simulink model "shuangxiangkaiguan"  (R2016b)
settings: Solver=ode23t  StartTime=0.0  StopTime=0.5  RelTol=1e-3
libraries: powerlib x31
settings Model: Creator=ChenNingke  LastModifiedBy=CNK

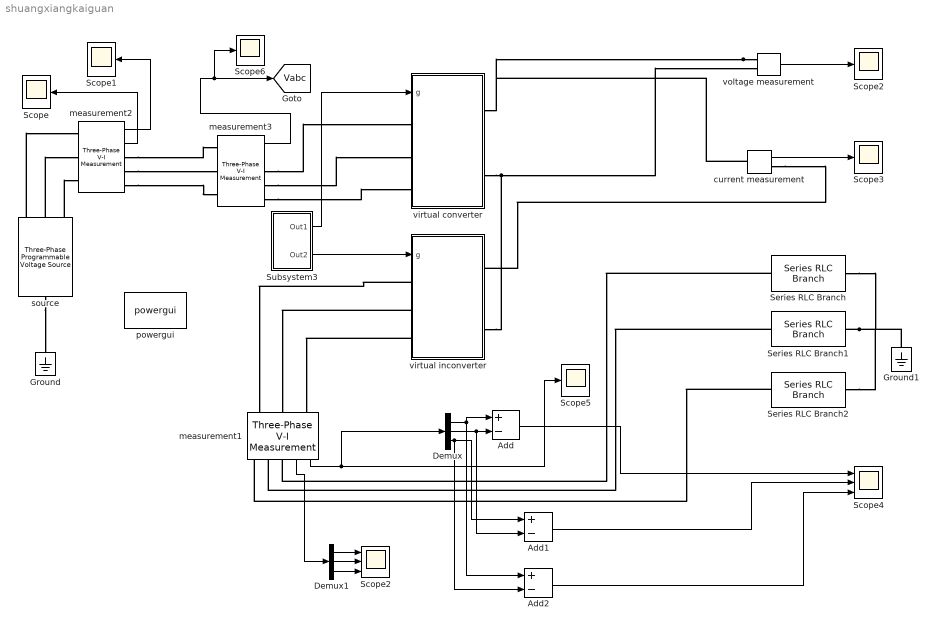
== system shuangxiangkaiguan ==
  Add : Sum  Inputs=+-
  Add1 : Sum  Inputs=+-
  Add2 : Sum  Inputs=+-
  Demux : Demux  Outputs=3
  Demux1 : Demux  Outputs=3
  Ground : powerlib/Elements/Ground  LConnTagsString=a
  Ground1 : powerlib/Elements/Ground  LConnTagsString=a
  Scope{,1,3,5..6} (5 alike) : Scope
  Scope2 : Scope  NumInputPorts=3
  "Scope2 " : Scope
  Scope4 : Scope  NumInputPorts=3
  Series RLC Branch : powerlib/Elements/Series RLC Branch  LConnTagsString=__new0  RConnTagsString=__new0  BranchType=RL  Resistance=5  Inductance=5e-3  SetiL0=off  InitialCurrent=0  Capacitance=1e-6  Setx0=off  InitialVoltage=0  Measurements=None
  Series RLC Branch1 : powerlib/Elements/Series RLC Branch  LConnTagsString=__new0  RConnTagsString=__new0  BranchType=RL  Resistance=5  Inductance=5e-3  SetiL0=off  InitialCurrent=0  Capacitance=1e-6  Setx0=off  InitialVoltage=0  Measurements=None
  Series RLC Branch2 : powerlib/Elements/Series RLC Branch  LConnTagsString=__new0  RConnTagsString=__new0  BranchType=RL  Resistance=5  Inductance=5e-3  SetiL0=off  InitialCurrent=0  Capacitance=1e-6  Setx0=off  InitialVoltage=0  Measurements=None
  Subsystem3 : Subsystem
  current measurement : powerlib/Measurements/Current Measurement  PhasorSimulation=off  OutputType=Complex  PSBequivalent=0
  measurement1 : powerlib/Measurements/Three-Phase V-I Measurement  VoltageMeasurement=phase-to-phase  SetLabelV=off  LabelV=Vabc  Vpu=off  VpuLL=off  CurrentMeasurement=yes  SetLabelI=off  LabelI=Iabc  Ipu=off  Pbase=100e6  Vbase=500e3  OutputType=Complex  PhasorSimulation=off  PSBequivalent=0
  measurement2 : powerlib/Measurements/Three-Phase V-I Measurement  VoltageMeasurement=phase-to-phase  SetLabelV=off  LabelV=Vabc  Vpu=off  VpuLL=off  CurrentMeasurement=yes  SetLabelI=off  LabelI=Iabc  Ipu=off  Pbase=100e6  Vbase=500e3  OutputType=Complex  PhasorSimulation=off  PSBequivalent=0
  measurement3 : powerlib/Measurements/Three-Phase V-I Measurement  VoltageMeasurement=phase-to-phase  SetLabelV=off  LabelV=Vabc  Vpu=off  VpuLL=off  CurrentMeasurement=yes  SetLabelI=off  LabelI=Iabc  Ipu=off  Pbase=100e6  Vbase=500e3  OutputType=Complex  PhasorSimulation=off  PSBequivalent=0
  powergui : powerlib/powergui  Priority=1  SimulationMode=Continuous  SolverType=Tustin  SampleTime=50e-6  frequency=60  SPID=off  DisableSnubberDevices=off  DisableRonSwitches=off  DisableVfSwitches=off  SwTol=0  DisplayEquations=off  Interpol=off  ExternalGateDelay=off  methode=off  Ts=10  FunctionMessages=off  echomessages=off  HookPort=off  EnableUseOfTLC=off  x0status=blocks  frequencyindice=0  Pbase=100e6  ErrMax=1e-4  Iterations=50  UnitsV=kV  UnitsW=MW  buscounter=0  RestoreLinks=warning  ResistiveCurrentMeasurement=off  Frange=[0:2:500]  Ylog=off  Xlog=on  ShowGrid=off  save=off  variable=ZData  structure=ScopeData6  ZoomFFT=off  StartTime=0.0  cycles=1  DisplayStyle=1  fundamental=600  FreqAxis=off  MaxFrequency=2000  frequencyindicesteady=1  RmsSteady=1  display=off
  source : powerlib/Electrical Sources/Three-Phase Programmable Voltage Source  PositiveSequence="[220  0 50]"  VariationEntity=None  VariationType=Table of time-amplitude pairs  VariationTypeAlt=Step  VariationStep=0.5  VariationRate=10  VariationMagnitude=0.3  VariationFrequency=2  VariationTiming=[1 2]  VariationPhaseA=off  Amplitudes=[1 0.8 1.2 1.0]  TimeValues=[0 0.1 0.15 0.2]  HarmonicGeneration=off  HarmonicA=[3 0.2 -25 0]  HarmonicB=[2 0.15 35 2]  Timing="[0.05  3]"  BusType=swing  Pref=0  Qref=0  Qmin=-inf  Qmax=inf
  virtual converter : Subsystem
  virtual inconverter : Subsystem
  voltage measurement : powerlib/Measurements/Voltage Measurement  PhasorSimulation=off  OutputType=Complex  PSBequivalent=0
  tag scope: Vabc=global
  wires:
  voltage measurement/1 -> "Scope2 "/1
  current measurement/1 -> Scope3/1
  measurement2/2 -> Scope/1
  measurement1/1 -> Demux/1, Scope5/1
  Subsystem3/2(Out2) -> virtual inconverter/1(g)
  Subsystem3/1(Out1) -> virtual converter/1(g)
  measurement2/1 -> Scope1/1
  Demux/1 -> Add2/1, Add/1
  Demux/2 -> Add1/2, Add/2
  Add/1 -> Scope4/1
  Demux/3 -> Add2/2, Add1/1
  Add1/1 -> Scope4/2
  Add2/1 -> Scope4/3
  measurement1/2 -> Demux1/1
  Demux1/1 -> Scope2/1
  Demux1/2 -> Scope2/2
  Demux1/3 -> Scope2/3
  measurement3/1 -> [Vabc], Scope6/1
  connections:
  voltage measurement/LConn1 -- current measurement/LConn1 -- virtual converter/RConn1
  virtual converter/RConn2 -- virtual inconverter/RConn2 -- voltage measurement/LConn2
  Series RLC Branch1/RConn1 -- Ground1/LConn1 -- Series RLC Branch/RConn1 -- Series RLC Branch2/RConn1
  Series RLC Branch1/LConn1 -- measurement1/RConn2
  current measurement/RConn1 -- virtual inconverter/RConn1
  Series RLC Branch/LConn1 -- measurement1/RConn1
  Series RLC Branch2/LConn1 -- measurement1/RConn3
  source/LConn1 -- Ground/LConn1
  virtual inconverter/LConn1 -- measurement1/LConn3
  virtual inconverter/LConn2 -- measurement1/LConn2
  virtual inconverter/LConn3 -- measurement1/LConn1
  source/RConn1 -- measurement2/LConn1
  source/RConn2 -- measurement2/LConn2
  source/RConn3 -- measurement2/LConn3
  measurement2/RConn1 -- measurement3/LConn1
  measurement2/RConn2 -- measurement3/LConn2
  measurement2/RConn3 -- measurement3/LConn3
  measurement3/RConn3 -- virtual converter/LConn3
  measurement3/RConn2 -- virtual converter/LConn2
  measurement3/RConn1 -- virtual converter/LConn1

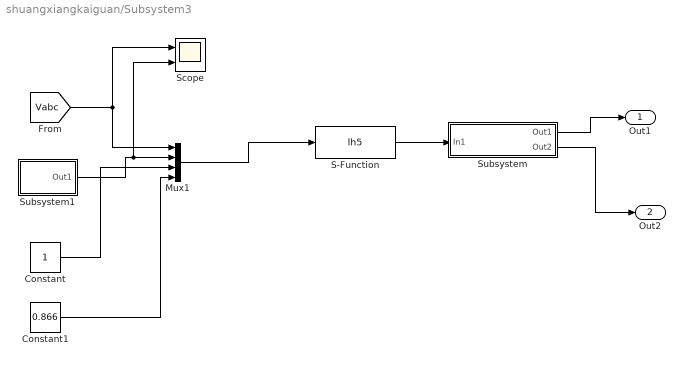
== system shuangxiangkaiguan/Subsystem3 ==
  Constant : Constant
  Constant1 : Constant  Value=0.866
  Mux1 : Mux
  S-Function : S-Function  FunctionName=lh5  SFunctionDeploymentMode=off  EnableBusSupport=off
  Scope : Scope  NumInputPorts=2
  Subsystem : Subsystem
  Subsystem1 : Subsystem
  Out1 : Outport
  Out2 : Outport  Port=2
  wires:
  [Vabc] -> Scope/1, Mux1/1
  Subsystem/1(Out1) -> Out1/1
  S-Function/1 -> Subsystem/1(In1)
  Subsystem1/1(Out1) -> Scope/2, Mux1/2
  Constant1/1 -> Mux1/4
  Constant/1 -> Mux1/3
  Subsystem/2(Out2) -> Out2/1
  Mux1/1 -> S-Function/1

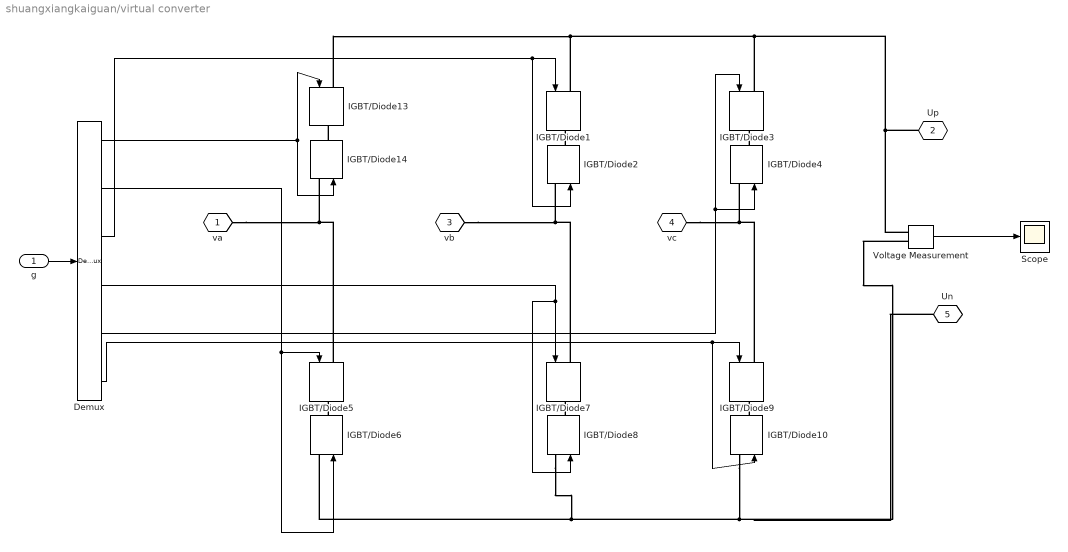
== system shuangxiangkaiguan/virtual converter ==
  g : Inport
  Demux : Demux  Outputs=6
  IGBT/Diode{1..10,13..14} (12 alike) : powerlib/Power Electronics/IGBT//Diode  Ron=1e-3  Rs=1e5  Cs=inf  Measurements=off
  Scope : Scope
  Voltage Measurement : powerlib/Measurements/Voltage Measurement  PhasorSimulation=off  OutputType=Complex  PSBequivalent=0
  va : PMIOPort  Tag=PMCPort  Port=1  Side=Left
  Up : PMIOPort  Tag=PMCPort  Port=2  Side=Right
  vb : PMIOPort  Tag=PMCPort  Port=3  Side=Left
  vc : PMIOPort  Tag=PMCPort  Port=4  Side=Left
  Un : PMIOPort  Tag=PMCPort  Port=5  Side=Right
  wires:
  g/1 -> Demux/1
  Demux/1 -> IGBT/Diode13/1, IGBT/Diode14/1
  Demux/3 -> IGBT/Diode1/1, IGBT/Diode2/1
  Demux/5 -> IGBT/Diode4/1, IGBT/Diode3/1
  Voltage Measurement/1 -> Scope/1
  Demux/2 -> IGBT/Diode5/1, IGBT/Diode6/1
  Demux/4 -> IGBT/Diode8/1, IGBT/Diode7/1
  Demux/6 -> IGBT/Diode10/1, IGBT/Diode9/1
  connections:
  va/RConn1 -- IGBT/Diode5/LConn1 -- IGBT/Diode14/LConn1
  vb/RConn1 -- IGBT/Diode7/LConn1 -- IGBT/Diode2/LConn1
  vc/RConn1 -- IGBT/Diode9/LConn1 -- IGBT/Diode4/LConn1
  Up/RConn1 -- Voltage Measurement/LConn1 -- IGBT/Diode1/LConn1 -- IGBT/Diode13/LConn1 -- IGBT/Diode3/LConn1
  Voltage Measurement/LConn2 -- Un/RConn1 -- IGBT/Diode10/LConn1 -- IGBT/Diode6/LConn1 -- IGBT/Diode8/LConn1
  IGBT/Diode14/RConn1 -- IGBT/Diode13/RConn1
  IGBT/Diode2/RConn1 -- IGBT/Diode1/RConn1
  IGBT/Diode4/RConn1 -- IGBT/Diode3/RConn1
  IGBT/Diode6/RConn1 -- IGBT/Diode5/RConn1
  IGBT/Diode8/RConn1 -- IGBT/Diode7/RConn1
  IGBT/Diode10/RConn1 -- IGBT/Diode9/RConn1

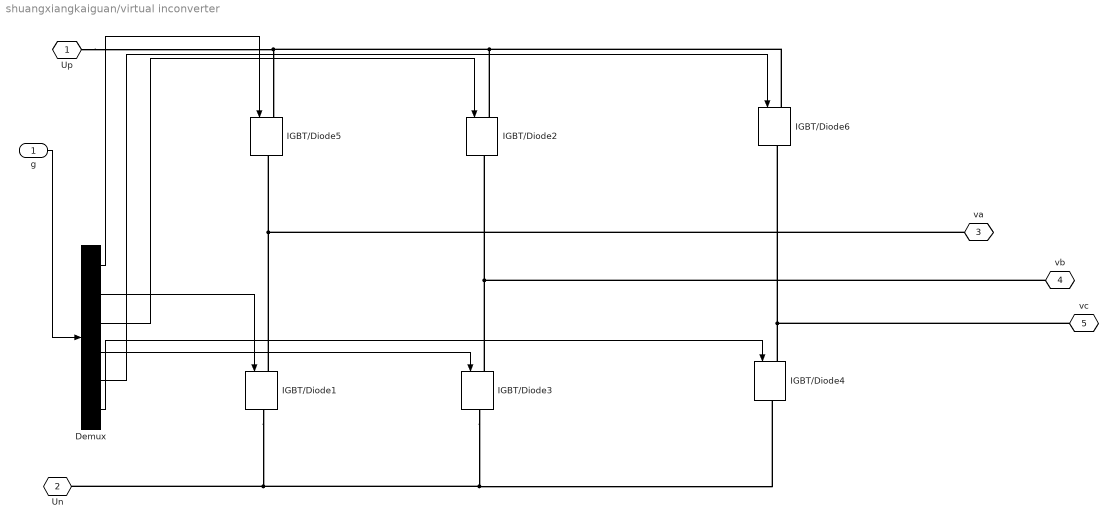
== system shuangxiangkaiguan/virtual inconverter ==
  g : Inport
  Demux : Demux  Outputs=6
  IGBT/Diode{1..6} (6 alike) : powerlib/Power Electronics/IGBT//Diode  Ron=1e-3  Rs=1e5  Cs=inf  Measurements=off
  Up : PMIOPort  Tag=PMCPort  Port=1  Side=Right
  Un : PMIOPort  Tag=PMCPort  Port=2  Side=Right
  va : PMIOPort  Tag=PMCPort  Port=3  Side=Left
  vb : PMIOPort  Tag=PMCPort  Port=4  Side=Left
  vc : PMIOPort  Tag=PMCPort  Port=5  Side=Left
  wires:
  g/1 -> Demux/1
  Demux/1 -> IGBT/Diode5/1
  Demux/3 -> IGBT/Diode2/1
  Demux/5 -> IGBT/Diode6/1
  Demux/6 -> IGBT/Diode4/1
  Demux/2 -> IGBT/Diode1/1
  Demux/4 -> IGBT/Diode3/1
  connections:
  vc/RConn1 -- IGBT/Diode6/RConn1 -- IGBT/Diode4/LConn1
  vb/RConn1 -- IGBT/Diode2/RConn1 -- IGBT/Diode3/LConn1
  va/RConn1 -- IGBT/Diode1/LConn1 -- IGBT/Diode5/RConn1
  Up/RConn1 -- IGBT/Diode2/LConn1 -- IGBT/Diode6/LConn1 -- IGBT/Diode5/LConn1
  Un/RConn1 -- IGBT/Diode4/RConn1 -- IGBT/Diode3/RConn1 -- IGBT/Diode1/RConn1

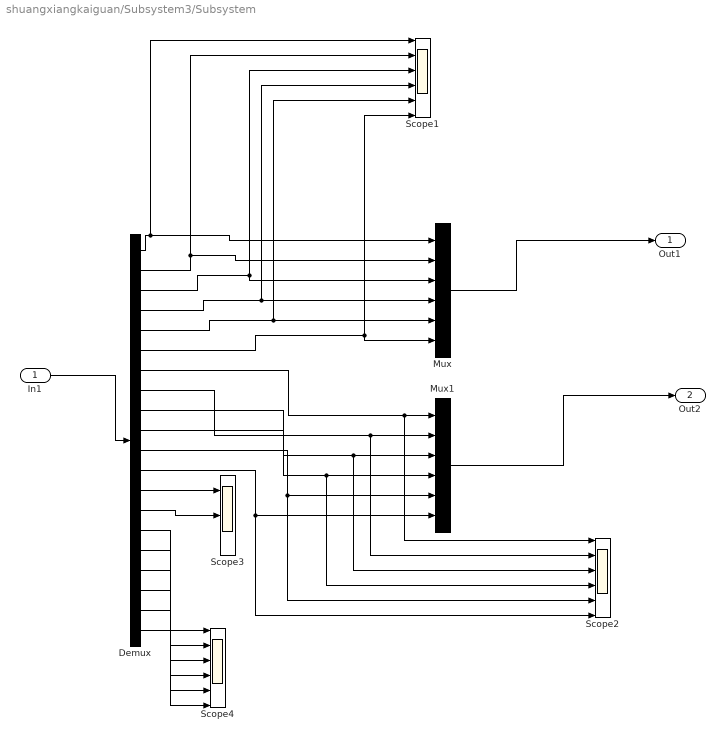
== system shuangxiangkaiguan/Subsystem3/Subsystem ==
  In1 : Inport
  Demux : Demux  Outputs=20
  Mux : Mux  Inputs=6
  Mux1 : Mux  Inputs=6
  Scope1 : Scope  NumInputPorts=6
  Scope2 : Scope  NumInputPorts=6
  Scope3 : Scope  NumInputPorts=3
  Scope4 : Scope  NumInputPorts=6
  Out1 : Outport
  Out2 : Outport  Port=2
  wires:
  In1/1 -> Demux/1
  Demux/1 -> Mux/1, Scope1/1
  Demux/2 -> Mux/2, Scope1/2
  Demux/3 -> Mux/3, Scope1/3
  Demux/4 -> Scope1/4, Mux/4
  Demux/5 -> Scope1/5, Mux/5
  Mux/1 -> Out1/1
  Demux/6 -> Mux/6, Scope1/6
  Demux/7 -> Scope2/1, Mux1/1
  Demux/8 -> Scope2/2, Mux1/2
  Demux/9 -> Scope2/3, Mux1/3
  Demux/10 -> Scope2/4, Mux1/4
  Demux/11 -> Scope2/5, Mux1/5
  Demux/12 -> Scope2/6, Mux1/6
  Mux1/1 -> Out2/1
  Demux/13 -> Scope3/1
  Demux/14 -> Scope3/2
  Demux/15 -> Scope4/1
  Demux/16 -> Scope4/2
  Demux/17 -> Scope4/3
  Demux/18 -> Scope4/4
  Demux/19 -> Scope4/5
  Demux/20 -> Scope4/6

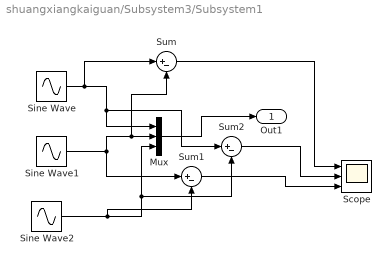
== system shuangxiangkaiguan/Subsystem3/Subsystem1 ==
  Mux : Mux  Inputs=3
  Scope : Scope  NumInputPorts=3
  Sine Wave : Sin  Amplitude=100  Frequency=10*2*pi  SampleTime=0
  Sine Wave1 : Sin  Amplitude=100  Frequency=10*2*pi  Phase=-2*pi/3  SampleTime=0
  Sine Wave2 : Sin  Amplitude=100  Frequency=10*2*pi  Phase=-4*pi/3  SampleTime=0
  Sum : Sum  Inputs=|+-
  Sum1 : Sum  Inputs=|+-
  Sum2 : Sum  Inputs=|+-
  Out1 : Outport
  wires:
  Sine Wave/1 -> Sum/1, Sum2/1, Mux/1
  Sine Wave1/1 -> Sum1/1, Sum/2, Mux/2
  Sine Wave2/1 -> Sum1/2, Sum2/2, Mux/3
  Mux/1 -> Out1/1
  Sum/1 -> Scope/1
  Sum1/1 -> Scope/3
  Sum2/1 -> Scope/2
